simulink library "LopesDevelopmentLibrary"  (R2015b)
settings: Solver=ode45  StartTime=0.0  StopTime=10.0  RelTol=1e-3
values from neighbouring files (symbols this model uses):
  d2r = @(d) d*(pi/180)    [LopesDevelopmentLibrary_LoadParameters.m]
  ts = LopesParams.ts    [LopesDevelopmentLibrary_LoadParameters.m]
undefined symbols (not defined in the file or in its folder): anyParameterChanged, DiscIntNeverNeededParam, gcbh, LAP, LHF, LKF, LopesParams, macaddr, mxpcnetworkconfig, mxpcrtudprx, mxpcrtudptx, patientParametersChanged, port, PX, PZ, RAP, RHF, RKF, SelectorLOPESInSize, StrideTime_s, Time
undefined symbols (not defined in the file): LopesParamsSendDataArrayLen
libraries: LopesDevelopmentLibrary x327, simulink x100, dspmtrx3 x49, xpciplib x6, xpcnetworkbufferlib x5, dspsigops x4, dspstat3 x3, xpcethernetlib x2, visionstatistics x2, xpcseriallib x2, LopesDevelopmentLibraryTest x1, nmc x1
(part 2 of 12)

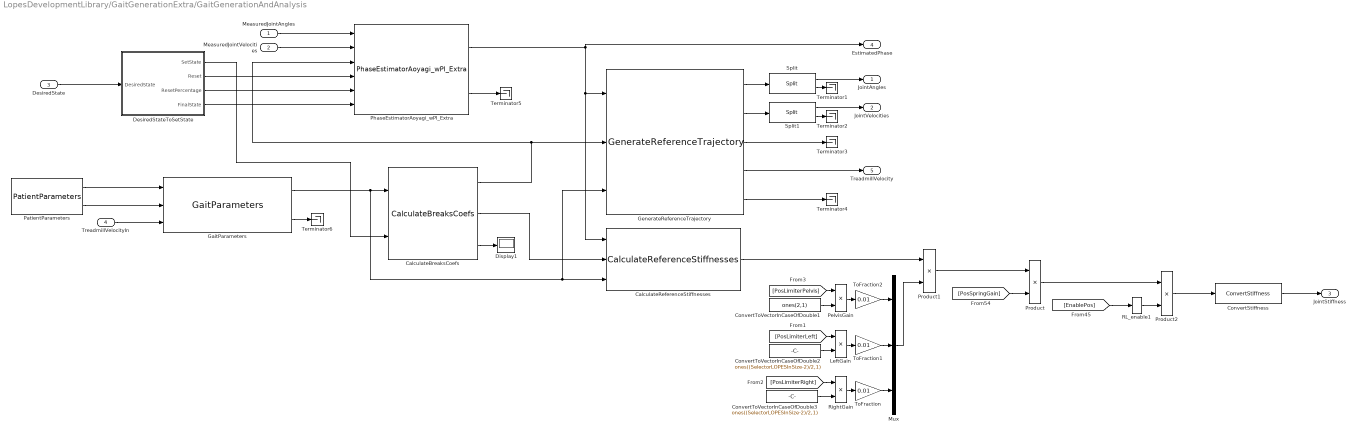
== system LopesDevelopmentLibrary/GaitGenerationExtra/GaitGenerationAndAnalysis ==
  MeasuredJointAngles : Inport
  MeasuredJointVelocities : Inport  Port=2
  DesiredState : Inport  Port=3
  TreadmillVelocityIn : Inport  Port=4
  CalculateBreaksCoefs : LopesDevelopmentLibrary/GaitGenerationExtra/CalculateBreaksCoefs
  CalculateReferenceStiffnesses : LopesDevelopmentLibrary/GaitGeneration/CalculateReferenceStiffnesses
  ConvertStiffness : LopesDevelopmentLibrary/GaitGeneration/ConvertStiffness
  ConvertToVectorInCaseOfDouble1 : Constant  Value=ones(2,1)
  ConvertToVectorInCaseOfDouble2 : Constant  Value=ones((SelectorLOPESInSize-2)/2,1)
  ConvertToVectorInCaseOfDouble3 : Constant  Value=ones((SelectorLOPESInSize-2)/2,1)
  DesiredStateToSetState : Subsystem
  Display1 : Display
  GaitParameters : LopesDevelopmentLibrary/GaitGenerationExtra/GaitParameters
  GenerateReferenceTrajectory : LopesDevelopmentLibrary/GaitGeneration/GenerateReferenceTrajectory
  LeftGain : Product
  Mux : Mux  Inputs=3
  PatientParameters : LopesDevelopmentLibrary/GaitGeneration/PatientParameters
      link override BodyLength_m: Value=1.88
      link override LowerLegLength_m: Value=0.44
      link override Mass_kg: Value=75
      link override UpperLegLength_m: Value=0.44
  PelvisGain : Product
  PhaseEstimatorAoyagi_wPI_Extra : LopesDevelopmentLibrary/GaitGenerationExtra/PhaseEstimatorAoyagi_wPI_Extra  Weights=[1.0, 0.1, 1.0, 0.1, 0.0, 0, 0.0, 0]  AoyagiFilterGain=0  AoyagiIntegralTimeConstant=5
  Product : Product
  Product1 : Product
  Product2 : Product
  RL_enable1 : nmc/RL_enable
  RightGain : Product
  Split : LopesDevelopmentLibrary/Various/Split
  Split1 : LopesDevelopmentLibrary/Various/Split
  Terminator{1..6} (6 alike) : Terminator
  ToFraction : Gain  Gain=0.01
  ToFraction1 : Gain  Gain=0.01
  ToFraction2 : Gain  Gain=0.01
  JointAngles : Outport
  JointVelocities : Outport  Port=2
  JointStiffness : Outport  Port=3
  EstimatedPhase : Outport  Port=4
  TreadmillVelocity : Outport  Port=5
  wires:
  DesiredStateToSetState/3(ResetPercentage) -> PhaseEstimatorAoyagi_wPI_Extra/5
  DesiredStateToSetState/2(Reset) -> PhaseEstimatorAoyagi_wPI_Extra/4
  DesiredState/1 -> DesiredStateToSetState/1(DesiredState)
  DesiredStateToSetState/1(SetState) -> CalculateBreaksCoefs/2
  CalculateBreaksCoefs/3 -> Display1/1
  CalculateBreaksCoefs/1 -> GenerateReferenceTrajectory/2, PhaseEstimatorAoyagi_wPI_Extra/3
  CalculateBreaksCoefs/2 -> CalculateReferenceStiffnesses/2
  PhaseEstimatorAoyagi_wPI_Extra/1 -> EstimatedPhase/1, GenerateReferenceTrajectory/1, CalculateReferenceStiffnesses/1
  GenerateReferenceTrajectory/1 -> Split/1
  Split/1 -> JointAngles/1
  Split/2 -> Terminator1/1
  GenerateReferenceTrajectory/5 -> Terminator4/1
  Split1/2 -> Terminator2/1
  PatientParameters/1 -> GaitParameters/1
  GenerateReferenceTrajectory/2 -> Split1/1
  Split1/1 -> JointVelocities/1
  MeasuredJointVelocities/1 -> PhaseEstimatorAoyagi_wPI_Extra/2
  MeasuredJointAngles/1 -> PhaseEstimatorAoyagi_wPI_Extra/1
  PhaseEstimatorAoyagi_wPI_Extra/2 -> Terminator5/1
  GenerateReferenceTrajectory/3 -> Terminator3/1
  PatientParameters/2 -> GaitParameters/2
  GaitParameters/2 -> Terminator6/1
  GaitParameters/1 -> CalculateBreaksCoefs/1, GenerateReferenceTrajectory/3, CalculateReferenceStiffnesses/3
  ConvertStiffness/1 -> JointStiffness/1
  CalculateReferenceStiffnesses/1 -> Product1/1
  [PosSpringGain] -> Product/2
  Product1/1 -> Product/1
  ConvertToVectorInCaseOfDouble1/1 -> PelvisGain/2
  [PosLimiterPelvis] -> PelvisGain/1
  [PosLimiterLeft] -> LeftGain/1
  ConvertToVectorInCaseOfDouble2/1 -> LeftGain/2
  [PosLimiterRight] -> RightGain/1
  ConvertToVectorInCaseOfDouble3/1 -> RightGain/2
  LeftGain/1 -> ToFraction1/1
  PelvisGain/1 -> ToFraction2/1
  Mux/1 -> Product1/2
  Product/1 -> Product2/1
  [EnablePos] -> RL_enable1/1
  RL_enable1/1 -> Product2/2
  Product2/1 -> ConvertStiffness/1
  RightGain/1 -> ToFraction/1
  ToFraction/1 -> Mux/3
  ToFraction1/1 -> Mux/2
  ToFraction2/1 -> Mux/1
  GenerateReferenceTrajectory/4 -> TreadmillVelocity/1
  DesiredStateToSetState/4(FinalState) -> PhaseEstimatorAoyagi_wPI_Extra/6
  TreadmillVelocityIn/1 -> GaitParameters/3

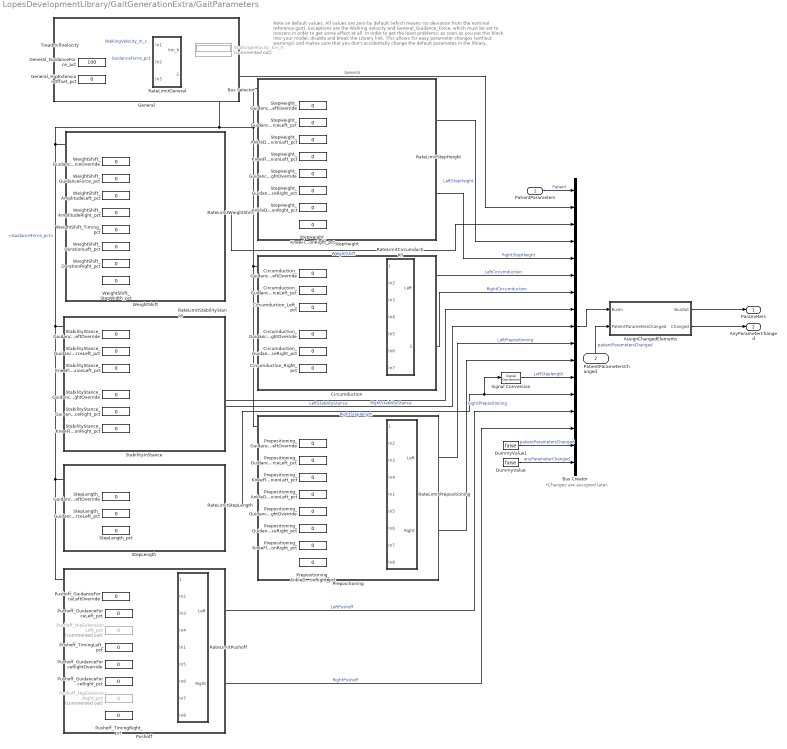
== system LopesDevelopmentLibrary/GaitGenerationExtra/GaitParameters ==
  note: Note on default values:
      | All values are zero by default (which means 'no deviation from the nominal reference gait).
      | Exceptions are the Walking velocity and General_Guidance_Force, which must be
      | set to nonzero in order to get some effect at all.
      |
      | In order to get the least problems: as soon as you put this block into your model, disable and
      | break the Library link. This allows for easy parameter changes (without warnings) and makes
      | sure that you don't accidentally change the default parametes in the library.
  note: *Changes are assigned later.
  PatientParameters : Inport
  PatientParametersChanged : Inport  Port=2
  TreadmillVelocity : Inport  Port=3
  AssignChangedElements : Subsystem
  Bus Creator : BusCreator  Inputs=17
  Bus Selector : BusSelector  OutputSignals=GuidanceForce_pct
  Circumduction : Subsystem
  Circumduction_GuidanceForceLeftOverride : Constant  Value=0  OutDataTypeStr=double
      settings: OpenFcn=|
      | b = get_param(gcb,'value');
      | if (strcmp(b,'1')),
      |   set_param (gcb,'value','0');
      | else
      |   set_param(gcb,'value','1');
      | end;
  Circumduction_GuidanceForceLeft_pct : Constant  Value=0
  Circumduction_GuidanceForceRightOverride : Constant  Value=0  OutDataTypeStr=double
      settings: OpenFcn=|
      | b = get_param(gcb,'value');
      | if (strcmp(b,'1')),
      |   set_param (gcb,'value','0');
      | else
      |   set_param(gcb,'value','1');
      | end;
  Circumduction_GuidanceForceRight_pct : Constant  Value=0
  Circumduction_Left_pct : Constant  Value=0
  Circumduction_Right_pct : Constant  Value=0
  DummyValue : Constant  Value=false  OutDataTypeStr=boolean
  DummyValue1 : Constant  Value=false
  General : Subsystem
  General_GuidanceForce_pct : Constant  Value=100
  General_HipExtensionOffset_pct : Constant  Value=0
  Prepositioning : Subsystem
  Prepositioning_AnkleDorsiFlexionLeft_pct : Constant  Value=0
  Prepositioning_AnkleDorsiFlexionRight_pct : Constant  Value=0
  Prepositioning_GuidanceForceLeftOverride : Constant  Value=0  OutDataTypeStr=double
      settings: OpenFcn=|
      | b = get_param(gcb,'value');
      | if (strcmp(b,'1')),
      |   set_param (gcb,'value','0');
      | else
      |   set_param(gcb,'value','1');
      | end;
  Prepositioning_GuidanceForceLeft_pct : Constant  Value=0
  Prepositioning_GuidanceForceRightOverride : Constant  Value=0  OutDataTypeStr=double
      settings: OpenFcn=|
      | b = get_param(gcb,'value');
      | if (strcmp(b,'1')),
      |   set_param (gcb,'value','0');
      | else
      |   set_param(gcb,'value','1');
      | end;
  Prepositioning_GuidanceForceRight_pct : Constant  Value=0
  Prepositioning_KneeFlexionLeft_pct : Constant  Value=0
  Prepositioning_KneeFlexionRight_pct : Constant  Value=0
  Pushoff : Subsystem
  Pushoff_GuidanceForceLeftOverride : Constant  Value=0  OutDataTypeStr=double
      settings: OpenFcn=|
      | b = get_param(gcb,'value');
      | if (strcmp(b,'1')),
      |   set_param (gcb,'value','0');
      | else
      |   set_param(gcb,'value','1');
      | end;
  Pushoff_GuidanceForceLeft_pct : Constant  Value=0
  Pushoff_GuidanceForceRightOverride : Constant  Value=0  OutDataTypeStr=double
      settings: OpenFcn=|
      | b = get_param(gcb,'value');
      | if (strcmp(b,'1')),
      |   set_param (gcb,'value','0');
      | else
      |   set_param(gcb,'value','1');
      | end;
  Pushoff_GuidanceForceRight_pct : Constant  Value=0
  Pushoff_HipExtensioRight_pct : Constant  Commented=on  Value=0
  Pushoff_HipExtensionLeft_pct : Constant  Commented=on  Value=0
  Pushoff_TimingLeft_pct : Constant  Value=0
  Pushoff_TimingRight_pct : Constant  Value=0
  RateLimitCircumduction : Subsystem
  RateLimitGeneral : Subsystem
  RateLimitPrepositioning : Subsystem
  RateLimitPushoff : Subsystem
  RateLimitStabilityStance : Subsystem
  RateLimitStepHeight : Subsystem
  RateLimitStepLength : Subsystem
  RateLimitWeightShift : Subsystem
  Signal Conversion : SignalConversion
  StabilityInStance : Subsystem
  StabilityStance_GuidanceForceLeftOverride : Constant  Value=0  OutDataTypeStr=double
      settings: OpenFcn=|
      | b = get_param(gcb,'value');
      | if (strcmp(b,'1')),
      |   set_param (gcb,'value','0');
      | else
      |   set_param(gcb,'value','1');
      | end;
  StabilityStance_GuidanceForceLeft_pct : Constant  Value=0
  StabilityStance_GuidanceForceRightOverride : Constant  Value=0  OutDataTypeStr=double
      settings: OpenFcn=|
      | b = get_param(gcb,'value');
      | if (strcmp(b,'1')),
      |   set_param (gcb,'value','0');
      | else
      |   set_param(gcb,'value','1');
      | end;
  StabilityStance_GuidanceForceRight_pct : Constant  Value=0
  StabilityStance_KneeFlexionLeft_pct : Constant  Value=0
  StabilityStance_KneeFlexionRight_pct : Constant  Value=0
  StepHeight : Subsystem
  StepHeight_AnkleDorsiflexionLeft_pct : Constant  Value=0
  StepHeight_AnkleDorsiflexionRight_pct : Constant  Value=0
  StepHeight_GuidanceForceLeftOverride : Constant  Value=0  OutDataTypeStr=double
      settings: OpenFcn=|
      | b = get_param(gcb,'value');
      | if (strcmp(b,'1')),
      |   set_param (gcb,'value','0');
      | else
      |   set_param(gcb,'value','1');
      | end;
  StepHeight_GuidanceForceLeft_pct : Constant  Value=0
  StepHeight_GuidanceForceRightOverride : Constant  Value=0  OutDataTypeStr=double
      settings: OpenFcn=|
      | b = get_param(gcb,'value');
      | if (strcmp(b,'1')),
      |   set_param (gcb,'value','0');
      | else
      |   set_param(gcb,'value','1');
      | end;
  StepHeight_GuidanceForceRight_pct : Constant  Value=0
  StepHeight_KneeFlexionLeft_pct : Constant  Value=0
  StepHeight_KneeFlexionRight_pct : Constant  Value=0
  StepLength : Subsystem
  StepLength_GuidanceForceLeftOverride : Constant  Value=0  OutDataTypeStr=double
      settings: OpenFcn=|
      | b = get_param(gcb,'value');
      | if (strcmp(b,'1')),
      |   set_param (gcb,'value','0');
      | else
      |   set_param(gcb,'value','1');
      | end;
  StepLength_GuidanceForceLeft_pct : Constant  Value=0
  StepLength_pct : Constant  Value=0
  WalkingVelocity_km_h : Display  Commented=on
  WeightShift : Subsystem
  WeightShift_AmplitudeLeft_pct : Constant  Value=0
  WeightShift_AmplitudeRight_pct : Constant  Value=0
  WeightShift_DurationLeft_pct : Constant  Value=0
  WeightShift_DurationRight_pct : Constant  Value=0
  WeightShift_GuidanceForceOverride : Constant  Value=0  OutDataTypeStr=double
      settings: OpenFcn=|
      | b = get_param(gcb,'value');
      | if (strcmp(b,'1')),
      |   set_param (gcb,'value','0');
      | else
      |   set_param(gcb,'value','1');
      | end;
  WeightShift_GuidanceForce_pct : Constant  Value=0
  WeightShift_StepWidth_pct : Constant  Value=0
  WeightShift_Timing_pct : Constant  Value=0
  Parameters : Outport
  AnyParameterChanged : Outport  Port=2
  wires:
  AssignChangedElements/1(BusOut) -> Parameters/1
  Signal Conversion/1 -> Bus Creator/12  "LeftSteplength"
  DummyValue1/1 -> Bus Creator/16  "patientParametersChanged"
  DummyValue/1 -> Bus Creator/17  "anyParameterChanged"
  RateLimitWeightShift/1(Out1) -> Bus Creator/3  "WeightShift"
  PatientParameters/1 -> Bus Creator/1  "Patient"
  RateLimitStepHeight/1(Left) -> Bus Creator/4  "LeftStepHeight"
  RateLimitStepHeight/2(Right) -> Bus Creator/5  "RightStepHeight"
  RateLimitStabilityStance/1(Left) -> Bus Creator/8  "LeftStabilityStance"
  RateLimitStabilityStance/2(Right) -> Bus Creator/9  "RightStabilityStance"
  RateLimitPrepositioning/1(Left) -> Bus Creator/10  "LeftPrepositioning"
  RateLimitPrepositioning/2(Right) -> Bus Creator/11  "RightPrepositioning"
  RateLimitStepLength/1(StepLength) -> Bus Creator/13, Signal Conversion/1  "RightSteplength"
  RateLimitCircumduction/1(Left) -> Bus Creator/6  "LeftCircumduction"
  RateLimitCircumduction/2(Right) -> Bus Creator/7  "RightCircumduction"
  WeightShift_GuidanceForceOverride/1 -> RateLimitWeightShift/2(In2)
  WeightShift_GuidanceForce_pct/1 -> RateLimitWeightShift/3(In3)
  WeightShift_AmplitudeLeft_pct/1 -> RateLimitWeightShift/4(In4)
  WeightShift_AmplitudeRight_pct/1 -> RateLimitWeightShift/5(In5)
  WeightShift_Timing_pct/1 -> RateLimitWeightShift/6(In6)
  WeightShift_DurationLeft_pct/1 -> RateLimitWeightShift/7(In7)
  WeightShift_DurationRight_pct/1 -> RateLimitWeightShift/8(In8)
  WeightShift_StepWidth_pct/1 -> RateLimitWeightShift/9(In9)
  StepHeight_GuidanceForceLeftOverride/1 -> RateLimitStepHeight/2(In2)
  StepHeight_GuidanceForceLeft_pct/1 -> RateLimitStepHeight/3(In3)
  StepHeight_KneeFlexionLeft_pct/1 -> RateLimitStepHeight/5(In4)
  StepHeight_GuidanceForceRightOverride/1 -> RateLimitStepHeight/6(In5)
  StepHeight_GuidanceForceRight_pct/1 -> RateLimitStepHeight/7(In6)
  StepHeight_KneeFlexionRight_pct/1 -> RateLimitStepHeight/9(In7)
  Circumduction_GuidanceForceLeftOverride/1 -> RateLimitCircumduction/2(In2)
  Circumduction_GuidanceForceLeft_pct/1 -> RateLimitCircumduction/3(In3)
  Circumduction_Left_pct/1 -> RateLimitCircumduction/4(In4)
  Circumduction_GuidanceForceRightOverride/1 -> RateLimitCircumduction/5(In5)
  Circumduction_GuidanceForceRight_pct/1 -> RateLimitCircumduction/6(In6)
  Circumduction_Right_pct/1 -> RateLimitCircumduction/7(In7)
  StabilityStance_GuidanceForceLeftOverride/1 -> RateLimitStabilityStance/2(In2)
  StabilityStance_GuidanceForceLeft_pct/1 -> RateLimitStabilityStance/3(In3)
  StabilityStance_KneeFlexionLeft_pct/1 -> RateLimitStabilityStance/4(In4)
  StabilityStance_GuidanceForceRightOverride/1 -> RateLimitStabilityStance/5(In5)
  StabilityStance_GuidanceForceRight_pct/1 -> RateLimitStabilityStance/6(In6)
  StabilityStance_KneeFlexionRight_pct/1 -> RateLimitStabilityStance/7(In7)
  Prepositioning_GuidanceForceLeftOverride/1 -> RateLimitPrepositioning/2(In2)
  Prepositioning_GuidanceForceLeft_pct/1 -> RateLimitPrepositioning/3(In3)
  Prepositioning_KneeFlexionLeft_pct/1 -> RateLimitPrepositioning/4(In4)
  Prepositioning_GuidanceForceRightOverride/1 -> RateLimitPrepositioning/6(In5)
  Prepositioning_GuidanceForceRight_pct/1 -> RateLimitPrepositioning/7(In6)
  Prepositioning_KneeFlexionRight_pct/1 -> RateLimitPrepositioning/8(In7)
  StepLength_GuidanceForceLeftOverride/1 -> RateLimitStepLength/2(In2)
  StepLength_GuidanceForceLeft_pct/1 -> RateLimitStepLength/3(In3)
  StepLength_pct/1 -> RateLimitStepLength/4(In4)
  Bus Selector/1 -> RateLimitStepHeight/1(GeneralGF), RateLimitPrepositioning/1(GeneralGF), RateLimitCircumduction/1(GeneralGF), RateLimitWeightShift/1(GeneralGF), RateLimitPushoff/1(GeneralGF), RateLimitStepLength/1(GeneralGF), RateLimitStabilityStance/1(GeneralGF)  "<GuidanceForce_pct>"
  RateLimitGeneral/2(General) -> Bus Creator/2, Bus Selector/1  "General"
  TreadmillVelocity/1 -> RateLimitGeneral/1(In1)  "WalkingVelocity_m_s"
  General_GuidanceForce_pct/1 -> RateLimitGeneral/2(In2)  "GuidanceForce_pct"
  General_HipExtensionOffset_pct/1 -> RateLimitGeneral/3(In3)
  RateLimitGeneral/1(km_h) -> WalkingVelocity_km_h/1
  Bus Creator/1 -> AssignChangedElements/1(BusIn)
  PatientParametersChanged/1 -> AssignChangedElements/2(PatientParametersChanged)  "patientParametersChanged"
  AssignChangedElements/2(Changed) -> AnyParameterChanged/1
  StepHeight_AnkleDorsiflexionLeft_pct/1 -> RateLimitStepHeight/4(In1)
  StepHeight_AnkleDorsiflexionRight_pct/1 -> RateLimitStepHeight/8(In8)
  Prepositioning_AnkleDorsiFlexionLeft_pct/1 -> RateLimitPrepositioning/5(In1)
  Prepositioning_AnkleDorsiFlexionRight_pct/1 -> RateLimitPrepositioning/9(In8)
  Pushoff_GuidanceForceLeft_pct/1 -> RateLimitPushoff/3(In3)
  Pushoff_HipExtensionLeft_pct/1 -> RateLimitPushoff/4(In4)
  Pushoff_GuidanceForceRightOverride/1 -> RateLimitPushoff/6(In5)
  Pushoff_GuidanceForceRight_pct/1 -> RateLimitPushoff/7(In6)
  Pushoff_HipExtensioRight_pct/1 -> RateLimitPushoff/8(In7)
  Pushoff_TimingLeft_pct/1 -> RateLimitPushoff/5(In1)
  Pushoff_TimingRight_pct/1 -> RateLimitPushoff/9(In8)
  RateLimitPushoff/1(Left) -> Bus Creator/14  "LeftPushoff"
  RateLimitPushoff/2(Right) -> Bus Creator/15  "RightPushoff"
  Pushoff_GuidanceForceLeftOverride/1 -> RateLimitPushoff/2(In2)

== system LopesDevelopmentLibrary/GaitGenerationExtra/PhaseEstimatorAoyagi_wPI_Extra ==
  note: This block is a phase estimator based on the paper by Aoyagi 2007. It consists of two parts:
      | -  a raw estimator which estimates the current phase simply based on the euclidean distance
      |    to each point on the trajectory (it returns the phase at which this distance is minimum), and
      | - a (sort-of-low-pass)-filter which generates a continuous and not-too-fast-changing output phase.
  MeasuredJointAngles : Inport
  MeasuredJointVelocities : Inport  Port=2
  BreaksCoefs : Inport  Port=3
  ResetHighActive : Inport  Port=4
  X0 : Inport  Port=5
  FinalState : Inport  Port=6
  Bus Selector : BusSelector  OutputSignals=StrideTime_s
  EstimatePhaseDirectlyAoyagi : Subsystem
  PhaseFilterAoyagi : Subsystem
  EstmiatedPhase_pct : Outport
  EstmiatedPhaseRate_pct_s : Outport  Port=2
  wires:
  FinalState/1 -> PhaseFilterAoyagi/5(FinalState)
  X0/1 -> PhaseFilterAoyagi/4(x0)
  MeasuredJointAngles/1 -> EstimatePhaseDirectlyAoyagi/1(MeasuredJointAngles)
  BreaksCoefs/1 -> EstimatePhaseDirectlyAoyagi/3(BreaksCoefs), Bus Selector/1
  MeasuredJointVelocities/1 -> EstimatePhaseDirectlyAoyagi/2(MeasuredJointVelocities)
  EstimatePhaseDirectlyAoyagi/1(EstimtatedPhaseUnfiltered) -> PhaseFilterAoyagi/1(EstimatedPhaseUnfiltered)
  Bus Selector/1 -> PhaseFilterAoyagi/2(ReferenceStrideTime)  "<StrideTime_s>"
  PhaseFilterAoyagi/1(EstimatedPhase) -> EstmiatedPhase_pct/1
  ResetHighActive/1 -> PhaseFilterAoyagi/3(ResetHighActive)
  PhaseFilterAoyagi/2(EstimatedPhaseRate) -> EstmiatedPhaseRate_pct_s/1

== system LopesDevelopmentLibrary/GaitGenerationExtra/VelocityHold ==
  SetState : Inport
  InputState : Inport  Port=2
  VeloIn : Inport  Port=3  OutDataTypeStr=double
  Compare To Constant5 : simulink/Logic and Bit Operations/Compare To Constant  Commented=on  relop===  const=3.0  OutDataTypeStr=boolean
  Compare To Constant6 : simulink/Logic and Bit Operations/Compare To Constant  Commented=on  relop=~=  const=301  OutDataTypeStr=boolean
  Compare To Constant7 : simulink/Logic and Bit Operations/Compare To Constant  Commented=on  relop=~=  const=302  OutDataTypeStr=boolean
  Compare To Constant8 : simulink/Logic and Bit Operations/Compare To Constant  Commented=on  relop=~=  const=401  OutDataTypeStr=boolean
  Compare To Constant9 : simulink/Logic and Bit Operations/Compare To Constant  Commented=on  relop=~=  const=402  OutDataTypeStr=boolean
  Constant : Constant  Value=0.25
  KeepSpeedUntillStopState : Gain  Commented=on  Gain=0.25
  Logical Operator2 : Logic  Commented=on  Inputs=4  AllPortsSameDT=off  OutDataTypeStr=boolean
  Logical Operator3 : Logic  Commented=on  AllPortsSameDT=off  OutDataTypeStr=boolean
  MATLAB Function : MATLAB Function  TreatAsAtomicUnit=on
      settings: MinAlgLoopOccurrences=on
  VeloOut : Outport  PortDimensions=1
  wires:
  SetState/1 -> MATLAB Function/2(SetState)
  Compare To Constant5/1 -> Logical Operator3/1
  Compare To Constant7/1 -> Logical Operator2/2
  ? -> Compare To Constant5/1
  Compare To Constant9/1 -> Logical Operator2/4
  Logical Operator2/1 -> Logical Operator3/2
  Compare To Constant6/1 -> Logical Operator2/1
  Compare To Constant8/1 -> Logical Operator2/3
  Logical Operator3/1 -> KeepSpeedUntillStopState/1
  ? -> Compare To Constant6/1
  ? -> Compare To Constant7/1
  ? -> Compare To Constant8/1
  ? -> Compare To Constant9/1
  InputState/1 -> MATLAB Function/1(InputState)
  Constant/1 -> MATLAB Function/4(LowerBound)
  MATLAB Function/1(VeloOut) -> VeloOut/1
  VeloIn/1 -> MATLAB Function/3(VeloIn)

== system LopesDevelopmentLibrary/GaitPhaseDetection/Gait Phase Detection with Wrapper ==
  note: Phase:
      | -2 -> Flight (or probably error)
      | -1 -> Error
      | 0 -> Error
      | 1 -> Double stance, left in front
      | 2 -> Right swing
      | 3 -> Double stance, right in front
      | 4 -> Left swing
  Cartesian Positions : Inport
  Treadmill : Inport  Port=2
  Data selection : Subsystem
  LeftLegWalking : Subsystem
  No speed detection : Subsystem
  Phase_selection : Subsystem
  RightLegWalking : Subsystem
  Smart derivative : Subsystem
  wAnkleConvert : Selector  InputPortWidth=33  IndexOptions=Index vector (dialog)  Indices=[1:12 19:27]  OutputSizes=1
  Phase : Outport
  wires:
  No speed detection/3(Right) -> Phase_selection/7(RightStop)
  No speed detection/2(Left) -> Phase_selection/6(LeftStop)
  Cartesian Positions/1 -> wAnkleConvert/1
  Phase_selection/1(Phase) -> Phase/1
  Smart derivative/4(ankle_y_r_dot) -> RightLegWalking/1(ankle_y_r_dot)
  Smart derivative/5(ankle_x_r_dot) -> RightLegWalking/2(ankle_x_r_dot)
  Smart derivative/6(angle_knee_r_dot) -> RightLegWalking/3(knee_angle_dot)
  Data selection/3(angle_knee_l) -> Smart derivative/3(angle_knee_l)
  Data selection/6(angle_knee_r) -> Smart derivative/6(angle_knee_r)
  Data selection/4(ankle_y_r) -> Smart derivative/4(ankle_y_r)
  Data selection/5(ankle_x_r) -> Phase_selection/5(ankle_x_r), Smart derivative/5(ankle_x_r)
  Data selection/2(ankle_x_l) -> Phase_selection/4(ankle_x_l), Smart derivative/2(ankle_x_l)
  Data selection/1(ankle_y_l) -> Smart derivative/1(ankle_y_l)
  Smart derivative/3(angle_knee_l_dot) -> LeftLegWalking/3(knee_angle_dot)
  Smart derivative/2(ankle_x_l_dot) -> LeftLegWalking/2(ankle_x_r_dot)
  Smart derivative/1(ankle_y_l_dot) -> LeftLegWalking/1(ankle_y_r_dot)
  Treadmill/1 -> Data selection/2(Treadmill), No speed detection/3(Treadmill)
  No speed detection/1(gaitSwitch) -> Phase_selection/3(Gait_switch)
  LeftLegWalking/1(Left) -> Phase_selection/1(LeftWalking)
  RightLegWalking/1(right) -> Phase_selection/2(RightWalking)
  Data selection/7(Treadmill speed) -> Smart derivative/7(treadmill speed), No speed detection/1(curVel), LeftLegWalking/4(belt_speed), RightLegWalking/4(belt_speed)
  wAnkleConvert/1 -> Data selection/1(Cart_pos), No speed detection/2(CartesianPositions)

== system LopesDevelopmentLibrary/GaitPhaseDetection/Gait Phase detection ==
  note: Phase:
      | -1 -> Error
      | 0 -> Error
      | 1 -> Double stance, left in front
      | 2 -> Right swing
      | 3 -> Double stance, right in front
      | 4 -> Left swing
  Cartesian Positions : Inport
  Treadmill : Inport  Port=2
  Data selection : Subsystem
  LeftLeg : Subsystem
  No speed detection : Subsystem
  Phase_selection : Subsystem
  RightLeg : Subsystem
  Smart derivative : Subsystem
  phase : Outport
  wires:
  Smart derivative/4(ankle_y_r_dot) -> RightLeg/1(ankle_y_r_dot)
  Smart derivative/5(ankle_x_r_dot) -> RightLeg/2(ankle_x_r_dot)
  Smart derivative/6(angle_knee_r_dot) -> RightLeg/3(knee_angle_dot)
  Data selection/7(Treadmill speed) -> Smart derivative/7(treadmill speed), No speed detection/1(curVel), LeftLeg/4(belt_speed), RightLeg/4(belt_speed)
  Data selection/3(angle_knee_l) -> Smart derivative/3(angle_knee_l)
  Data selection/6(angle_knee_r) -> Smart derivative/6(angle_knee_r)
  Data selection/4(ankle_y_r) -> Smart derivative/4(ankle_y_r)
  Data selection/5(ankle_x_r) -> Smart derivative/5(ankle_x_r), Phase_selection/5(ankle_x_r)
  Data selection/2(ankle_x_l) -> Smart derivative/2(ankle_x_l), Phase_selection/4(ankle_x_l)
  Data selection/1(ankle_y_l) -> Smart derivative/1(ankle_y_l)
  Smart derivative/3(angle_knee_l_dot) -> LeftLeg/3(knee_theta_l_dot)
  Smart derivative/2(ankle_x_l_dot) -> LeftLeg/2(ankle_x_l_dot)
  Smart derivative/1(ankle_y_l_dot) -> LeftLeg/1(ankle_y_l_dot)
  Treadmill/1 -> Data selection/2(Treadmill)
  Cartesian Positions/1 -> Data selection/1(Cart_pos)
  Phase_selection/1(Phase) -> phase/1
  No speed detection/1(gaitSwitch) -> Phase_selection/3(Gait_switch)
  LeftLeg/1(left) -> Phase_selection/1(Left)
  RightLeg/1(right) -> Phase_selection/2(Right)

== system LopesDevelopmentLibrary/Mindwalker/Mindwalker_AdaptiveTreadmillVelocity ==
  note: The treadmill should, on average, have the same velocity as the resulting
      | walking velocity (keeping in mind that the user regularly stands still). We do this
      | by making the treadmill velocity a function of PX: the more to the front the
      | user is, the faster the treadmill goes. In order to get everything smooth, we also use
      | a (very low frequency) low pas filter. The aim is that, you'll never be pushed against the
      | back stop of PX by the treadmill if you stand still. Therefore, we have a 'dead zone'
      | close to the back stop, where the treadmill is off. Outside the dead zone, the
      | velocity is linear with PX, up to a maximum of V_treadmill_max, which is the velocity
      | if you'd initiate steps as fast as possible. The boundary between dead zone and linear zone is
      | called 'Threshold'.
      |
      | Note that the (current) range of motion for PX is -0.18...0.17 m.
  Lopes_ModelPos : Inport
  State : Inport  Port=2
  CalculateThreshold : Sum
  CompareAny : LopesDevelopmentLibrary/Various/CompareAny  values=[2,3,5,6,8,9]
  Data Type Conversion : DataTypeConversion  OutDataTypeStr=double
  Demux : Demux  Outputs=2
  Divide : Product  Inputs=*/
  GetPX : Selector  InputPortWidth=11  IndexOptions=Index vector (dialog)  Indices=1  OutputSizes=1
  Product : Product  RndMeth=Zero
  Product1 : Product  RndMeth=Zero
  RangeOfMotionPX_m : Constant  Value=[-0.18,0.17]
  Saturation : Saturate  UpperLimit=5  LowerLimit=0
  SecondOrderLowPassFilter : LopesDevelopmentLibrary/Various/SecondOrderLowPassFilter  w=10*(2*pi)  z=1
  Subtract : Sum  Inputs=+-
  Subtract1 : Sum  Inputs=+-
  V_treadmill_max : Constant  Value=0.5
  deadZone_m : Constant  Value=0.01
  TreadmillVelocity : Outport
  wires:
  Saturation/1 -> TreadmillVelocity/1
  Data Type Conversion/1 -> Product1/2
  State/1 -> CompareAny/1
  CompareAny/1 -> Data Type Conversion/1
  Product1/1 -> Product/2
  SecondOrderLowPassFilter/1 -> Saturation/1
  Product/1 -> SecondOrderLowPassFilter/1
  V_treadmill_max/1 -> Product1/1
  Divide/1 -> Product/1
  Subtract1/1 -> Divide/2
  Subtract/1 -> Divide/1
  Lopes_ModelPos/1 -> GetPX/1
  CalculateThreshold/1 -> Subtract1/2, Subtract/2
  Demux/1 -> CalculateThreshold/2
  deadZone_m/1 -> CalculateThreshold/1
  Demux/2 -> Subtract1/1
  RangeOfMotionPX_m/1 -> Demux/1
  GetPX/1 -> Subtract/1

== system LopesDevelopmentLibrary/Mindwalker/Mindwalker_Lopes_Conversion ==
  note: Visualization works only in normal
      | simulation mode (not when using xPC Target)
  Lopes_ModelPos : Inport
  Lopes_ModelVel : Inport  Port=2
  MW_SpringPositions : Inport  Port=3
  MW_SpringVelocities : Inport  Port=4
  MW_SpringStiffnesses : Inport  Port=5
  MW_BiasForces : Inport  Port=6
  CalculateForceOnTorso : Subsystem
  EnableVisualization : Constant  OutDataTypeStr=double
      settings: OpenFcn=|
      | b = get_param(gcb,'value');
      | if (strcmp(b,'1')),
      |   set_param (gcb,'value','0');
      | else
      |   set_param(gcb,'value','1');
      | end;
  ITorso_kgm2 : Constant  Value=6.73
  LopesToMWPosition : Subsystem
  LopesToMWVelocity : Subsystem
  MWToLopesPosition : Subsystem
  MWToLopesVelocity : Subsystem
  Mux1 : Mux  Inputs=2
  Mux2 : Mux  Inputs=2
  TorsoDynamics : Subsystem
  VisualizeStickFigure : Subsystem  Commented=on
  Zeros : Constant  Value=[0;0]
  Zeros1 : Constant  Value=[0,0]
  Lopes_SpringPositions : Outport
  Lopes_SpringVelocities : Outport  Port=2
  Lopes_SpringStiffnesses : Outport  Port=3
  Lopes_BiasForces : Outport  Port=4
  MW_ModelPos : Outport  Port=5
  MW_ModelVel : Outport  Port=6
  wires:
  LopesToMWVelocity/1(MW_Joints) -> MW_ModelVel/1
  LopesToMWPosition/1(MW_Joints) -> MW_ModelPos/1
  CalculateForceOnTorso/1(ForceOnTorso) -> TorsoDynamics/1(Force)
  Lopes_ModelVel/1 -> LopesToMWVelocity/1(Lopes_Joints), CalculateForceOnTorso/6(Lopes_ModelVel)
  TorsoDynamics/2(TorsoFlexionVelocity) -> MWToLopesVelocity/2(TorsoValue), LopesToMWVelocity/2(TorsoValue)
  TorsoDynamics/1(TorsoFlexion) -> VisualizeStickFigure/1(TorsoFlexion), MWToLopesPosition/2(TorsoValue), LopesToMWPosition/2(TorsoValue)
  EnableVisualization/1 -> VisualizeStickFigure/3(Enable)
  MW_BiasForces/1 -> CalculateForceOnTorso/4(MW_BiasForces), Mux1/2
  Mux2/1 -> Lopes_SpringStiffnesses/1
  MW_SpringPositions/1 -> MWToLopesPosition/1(RelativeJoints)
  Zeros/1 -> Mux1/1
  Zeros1/1 -> Mux2/1
  Lopes_ModelPos/1 -> CalculateForceOnTorso/5(Lopes_ModelPos), VisualizeStickFigure/2(Lopes_ModelPos), LopesToMWPosition/1(Lopes_Joints)
  MWToLopesPosition/1(AbsoluteJoints) -> Lopes_SpringPositions/1, CalculateForceOnTorso/1(MW_SpringPositions)
  MWToLopesVelocity/1(AbsoluteJoints) -> Lopes_SpringVelocities/1, CalculateForceOnTorso/2(MW_SpringVelocities)
  MW_SpringVelocities/1 -> MWToLopesVelocity/1(RelativeJoints)
  ITorso_kgm2/1 -> CalculateForceOnTorso/7(Inertia), TorsoDynamics/2(Inertia)
  MW_SpringStiffnesses/1 -> Mux2/2, CalculateForceOnTorso/3(MW_SpringStiffness)
  Mux1/1 -> Lopes_BiasForces/1

== system LopesDevelopmentLibrary/Robot control blocks/FromLopes ==
  note: These gains are here to have a common
      | location from where we can obtain the
      | values, for example by using the
      | xpc module in Python.
  note: This block periodically (with a period of Decimation*sampletime) requests joint angle
      | data from the LLC. This happens by sending a request string, and receiving the
      | response from the LLC. Note that it may be the case that it will receive old data
      | (this happens when the LLC was not fast enough to process the request, which may happen
      | if the receive block is executed very shortly after the sending block). So, it could be
      | that the received data is (Decimation*sampletime) seconds old.
  note: If ErrorValue is zero, everything is fine. If nonzero,
      | refer to the code inside ParseString to see
      | what's wrong.
  AnalogInput_ : Concatenate  NumInputs=1
  CartesianPositions_ : Concatenate  NumInputs=1
  Decimation : LopesDevelopmentLibrary/Various/Decimation
  EnableAnalogInput : Constant  OutDataTypeStr=double
      settings: OpenFcn=|
      | b = get_param(gcb,'value');
      | if (strcmp(b,'1')),
      |   set_param (gcb,'value','0');
      | else
      |   set_param(gcb,'value','1');
      | end;
  EnableDebugStringsInMatlab : Constant  Value=0  OutDataTypeStr=double
      settings: OpenFcn=|
      | b = get_param(gcb,'value');
      | if (strcmp(b,'1')),
      |   set_param (gcb,'value','0');
      | else
      |   set_param(gcb,'value','1');
      | end;
  ErrorValue : Display  Commented=on
      settings: AttributesFormatString=%<Tag>
  GenerateString : Subsystem
  LLCReceiveUDPChannel2 : LopesDevelopmentLibrary/BlocksForInternalUse/LLC Communication/LLCReceiveUDP  port=LopesParams.Communication.channel2ReceivePort
  LLCSendUDPChannel2 : LopesDevelopmentLibrary/BlocksForInternalUse/LLC Communication/LLCSendUDP  port=LopesParams.Communication.channel2SendPort
  Logical Operator : Logic  AllPortsSameDT=off  OutDataTypeStr=boolean
  Logical Operator1 : Logic  AllPortsSameDT=off  OutDataTypeStr=boolean
  MeasForces_ : Concatenate  NumInputs=1
  MeasPos_ : Concatenate  NumInputs=1
  ModelAcc_ : Concatenate  NumInputs=1
  ModelPos_ : Concatenate  NumInputs=1
  ModelVel_ : Concatenate  NumInputs=1
  One : Constant
  ParseError_ : Concatenate  NumInputs=1
  ParseString : Subsystem
  PreRecv : Constant  Value=uint8(['FromLopes Recv: '])
  PreSend : Constant  Value=uint8(['FromLopes Send: '])
  ShowStringInMatlabConsole : MATLAB Function  TreatAsAtomicUnit=on
  ShowStringInMatlabConsole1 : MATLAB Function  TreatAsAtomicUnit=on
  Treadmill_ : Concatenate  NumInputs=1
  ~Debug : Subsystem
      mask Display: disp('')
  Error : Outport
  ModelPos : Outport  Port=2
  ModelVel : Outport  Port=3
  ModelAcc : Outport  Port=4
  MeasPos : Outport  Port=5
  MeasForces : Outport  Port=6
  CartesianPositions : Outport  Port=7
  Treadmill : Outport  Port=8
  AnalogInput : Outport  Port=9
  wires:
  AnalogInput_/1 -> AnalogInput/1
  ParseString/9(AnalogInput) -> AnalogInput_/1
  EnableAnalogInput/1 -> GenerateString/1(EnableAnaloginput)
  PreSend/1 -> ShowStringInMatlabConsole1/3(pre)
  GenerateString/2(s_len) -> ShowStringInMatlabConsole1/2(len), LLCSendUDPChannel2/2
  GenerateString/1(s) -> ShowStringInMatlabConsole1/1(stringArray), LLCSendUDPChannel2/1
  Treadmill_/1 -> Treadmill/1
  CartesianPositions_/1 -> CartesianPositions/1
  MeasForces_/1 -> MeasForces/1
  MeasPos_/1 -> MeasPos/1
  ModelAcc_/1 -> ModelAcc/1
  ModelVel_/1 -> ModelVel/1
  ModelPos_/1 -> ModelPos/1
  ParseError_/1 -> ErrorValue/1, Error/1
  ParseString/8(Treadmill) -> Treadmill_/1
  ParseString/7(ModelCartPos) -> CartesianPositions_/1
  ParseString/6(MeasForce) -> MeasForces_/1
  ParseString/4(ModelAcc) -> ModelAcc_/1
  ParseString/3(ModelVel) -> ModelVel_/1
  ParseString/2(ModelPos) -> ModelPos_/1
  ParseString/1(ParseError) -> ParseError_/1
  ParseString/5(MeasPos) -> MeasPos_/1
  Decimation/1 -> Logical Operator/2, LLCSendUDPChannel2/Enable, GenerateString/Enable
  PreRecv/1 -> ShowStringInMatlabConsole/3(pre)
  LLCReceiveUDPChannel2/2 -> ParseString/2(In2), ShowStringInMatlabConsole/2(len)
  LLCReceiveUDPChannel2/1 -> ShowStringInMatlabConsole/1(stringArray), ParseString/1(In1)
  EnableDebugStringsInMatlab/1 -> Logical Operator1/1, Logical Operator/1
  Logical Operator/1 -> ShowStringInMatlabConsole1/4(enable)
  One/1 -> ParseString/Enable, LLCReceiveUDPChannel2/Enable, Logical Operator1/2
  Logical Operator1/1 -> ShowStringInMatlabConsole/4(enable)

== system LopesDevelopmentLibrary/Robot control blocks/GeneralLopes ==
  note: 0: off
      | 1: init
      | 2: home
      | 3: stop
      | 4: position
      | 5: force
  note: 0: off
      | 1: init
      | 2: home
      | 3: stop
      | 4: position
      | 5: force
  note: This block periodically (with a period of Decimation*sampletime) checks the state of Lopes.
      | Additionally, it allows the user to request a state ('off', 'init', 'home', 'stop','position', 'force').
      | This happens by sending a request string, and receiving the
      | response from the LLC. Note that it may be the case that it will receive old data
      | (this happens when the LLC was not fast enough to process the request, which may happen
      | if the receive block is executed very shortly after the sending block).
  note: These blocks are here to have a common
      | location from where we can obtain the
      | values, for example by using the
      | xpc module in Python.
  note: You can leave this input
      | unconnected to get the
      | default inertia
  note: Set to 0 to disable
      | the watchdog
  note: -1: No message received (note that if decimation~=1, this happens  often)
      | 0: No error
      | 1: Error
  note: Temporarily removed input
      | SegmentInertia because it
      | doesn't affect the used inertia
      | (LLC uses CartesianInertia by default)
  DesiredState : Inport
  AnyMessageWasReceived : Subsystem
  Bus Creator : BusCreator  Inputs=6
  Decimation : LopesDevelopmentLibrary/Various/Decimation
      settings: Decimation=10
  EnableDebugStringsInMatlab : Constant  Value=0  OutDataTypeStr=double
      settings: OpenFcn=|
      | b = get_param(gcb,'value');
      | if (strcmp(b,'1')),
      |   set_param (gcb,'value','0');
      | else
      |   set_param(gcb,'value','1');
      | end;
  ErrorDisplay : Display  Commented=on
      settings: AttributesFormatString=%<Tag>
  GenerateString : Subsystem
  Ground : Ground
  LLC Network Configuration : LopesDevelopmentLibrary/BlocksForInternalUse/LLC Communication/LLC Network Configuration
  LLCReceiveUDPChannel1 : LopesDevelopmentLibrary/BlocksForInternalUse/LLC Communication/LLCReceiveUDP  port=LopesParams.Communication.channel1ReceivePort
  LLCSendUDPChannel1 : LopesDevelopmentLibrary/BlocksForInternalUse/LLC Communication/LLCSendUDP  port=LopesParams.Communication.channel1SendPort
  Logical Operator : Logic  AllPortsSameDT=off  OutDataTypeStr=boolean
  Logical Operator1 : Logic  AllPortsSameDT=off  OutDataTypeStr=boolean
  One : Constant
  ParseString : Subsystem
  PreRecv : Constant  Value=uint8(['General Recv: '])
  PreSend : Constant  Value=uint8(['General Send: '])
  ShowStringInMatlabConsole : MATLAB Function  TreatAsAtomicUnit=on
  ShowStringInMatlabConsole1 : MATLAB Function  TreatAsAtomicUnit=on
  WatchdogTimeout_ms : Constant  Value=500
  error_ : Concatenate  NumInputs=1
  isCabinetBlueButtonPressed_ : Concatenate  NumInputs=1
  isInitOk_ : Concatenate  NumInputs=1
  isMotorsOk_ : Concatenate  NumInputs=1
  isPatientDefined_ : Concatenate  NumInputs=1
  isTreadmillEmpty_ : Concatenate  NumInputs=1
  llcState : Display  Commented=on
      settings: AttributesFormatString=%<Tag>
  llcState_ : Concatenate  NumInputs=1
  ~Debug : Subsystem
      mask Display: disp('')
  Error : Outport
  LopesStatus : Outport  Port=2
  wires:
  AnyMessageWasReceived/1(Out1) -> GenerateString/4(AnyMessageWasReceivedByLLC)
  WatchdogTimeout_ms/1 -> GenerateString/3(WatchdogTimeout_ms)
  Ground/1 -> GenerateString/2(SegmentInertia)
  PreRecv/1 -> ShowStringInMatlabConsole1/3(pre)
  LLCReceiveUDPChannel1/2 -> ShowStringInMatlabConsole1/2(len), ParseString/2(s_len)
  LLCReceiveUDPChannel1/1 -> ShowStringInMatlabConsole1/1(stringArray), ParseString/1(s)
  PreSend/1 -> ShowStringInMatlabConsole/3(pre)
  Decimation/1 -> Logical Operator/2, GenerateString/Enable, LLCSendUDPChannel1/Enable
  ParseString/4(isInitOk) -> isInitOk_/1
  ParseString/7(isPatientDefined) -> isPatientDefined_/1
  ParseString/1(isParseException) -> AnyMessageWasReceived/1(In1), ErrorDisplay/1, error_/1
  ParseString/5(isMotorsOk) -> isMotorsOk_/1
  ParseString/2(llcState) -> llcState_/1
  ParseString/6(isTreadmillEmpty) -> isTreadmillEmpty_/1
  isPatientDefined_/1 -> Bus Creator/6  "isPatientDefined"
  isTreadmillEmpty_/1 -> Bus Creator/5  "isTreadmillEmpty"
  Bus Creator/1 -> LopesStatus/1
  isInitOk_/1 -> Bus Creator/3  "isInitOk"
  llcState_/1 -> llcState/1, Bus Creator/1  "llcState"
  isMotorsOk_/1 -> Bus Creator/4  "isMotorsOk"
  isCabinetBlueButtonPressed_/1 -> Bus Creator/2  "isCabinetBlueButtonPressed"
  GenerateString/2(s_len) -> LLCSendUDPChannel1/2, ShowStringInMatlabConsole/2(len)
  GenerateString/1(s) -> LLCSendUDPChannel1/1, ShowStringInMatlabConsole/1(stringArray)
  DesiredState/1 -> GenerateString/1(DesiredState)
  EnableDebugStringsInMatlab/1 -> Logical Operator1/1, Logical Operator/1
  Logical Operator/1 -> ShowStringInMatlabConsole/4(enable)
  One/1 -> LLCReceiveUDPChannel1/Enable, Logical Operator1/2, ParseString/Enable
  ParseString/3(isBlueCabinetButtonPressed) -> isCabinetBlueButtonPressed_/1
  Logical Operator1/1 -> ShowStringInMatlabConsole1/4(enable)
  error_/1 -> Error/1

== system LopesDevelopmentLibrary/Robot control blocks/RS232SyncBox ==
  note: You can use this block to send or receive (sync) pulses using the second RS232
      | (on the silver embedded PC's, this is the RS232 on the side where also keyboard
      | and network connectors are). This block was made to work together with the Lopes Sync Box.
      |
      | The input isSend determines the behaviour of this block:
      |
      | isSend==True (nonzero):
      | The system will send the (bool-typecast) of In to the DTR line of the RS232.
      | The output Out is made equal to In (such that, both for sending and receiving, Out reflects the sync pulse).
      |
      | isSend==False (zero):
      | The system sets the DTR and RTS such that the Sync box is configured for input;
      | then the output Out is set to what is coming in on the CTS input of the RS232. The value
      | of input In is ignored.
      |
      | This block was designed to be used with the Lopes-Sync Box. This box was constructed such
      | that for using the input on the box, DTR should be 0 and RTS should be 1.
  isSend : Inport
  In : Inport  Port=2
  Compare To Zero1 : simulink/Logic and Bit Operations/Compare To Zero  relop=~=  OutDataTypeStr=boolean
  DTR_Read : Constant  Value=0
  DTR_Send : DataTypeConversion  OutDataTypeStr=double
  Modem Control : xpcseriallib/Mainboard/Modem Control  rts=on  dtr=on  config=Com2  addr=0x3f8
  Modem Status : xpcseriallib/Mainboard/Modem Status  cts=on  dsr=off  ring=off  dcd=off  sampletime=HLCParams.ts  config=Com2  addr=0x3f8
  RTS_Read : Constant
  RTS_Send : Constant  Value=0
  Switch : Switch  Criteria=u2 ~= 0
  Switch1 : Switch  Criteria=u2 ~= 0
  Switch2 : Switch  Criteria=u2 ~= 0
  Out : Outport
  wires:
  isSend/1 -> Switch/2, Switch2/2, Switch1/2
  DTR_Send/1 -> Switch/1, Switch2/1
  Modem Status/1 -> Switch/3
  Switch/1 -> Out/1
  In/1 -> Compare To Zero1/1
  Switch2/1 -> Modem Control/2
  DTR_Read/1 -> Switch2/3
  Compare To Zero1/1 -> DTR_Send/1
  Switch1/1 -> Modem Control/1
  RTS_Send/1 -> Switch1/1
  RTS_Read/1 -> Switch1/3

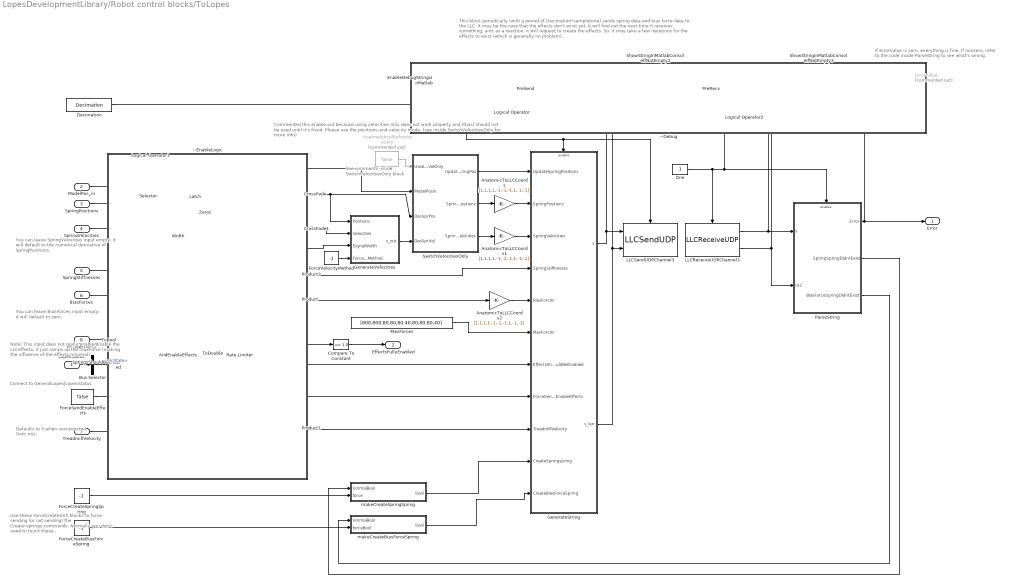
== system LopesDevelopmentLibrary/Robot control blocks/ToLopes ==
  note: You can leave BiasForces
      | input empty; it will default to zero.
  note: This block periodically (with a period of Decimation*sampletime) sends spring data and bias force
      | data to the LLC.
      | It may be the case that the effects don't exist yet. It will find out the next time it receives something, and,
      | as a reaction, it will request to create the effects. So, it may take a few iterations for the effects
      | to exist (which is generally no problem).
  note: If ErrorValue is zero, everything is fine. If nonzero,
      | refer to the code inside ParseString to see
      | what's wrong.
  note: Use these ForceCreateXXX
      | blocks to force sending (or not sending)
      | the Create-springs-commands.
      | Normally you don't need to touch these..
  note: You can leave SpringVelocities
      | input empty; it will default to the
      | numerical derivative of SpringPositions.
  note: Note: This input does not really enable/disable
      | the LLCeffects; it just ramps up the maxForce
      | (making the influence of the effects minimal)
  note: Connect to GeneralLopes|LopesStatus
  note: Defaults to 0 when unconnected.
      | Unit: m/s.
  note: See comments inside
      | SwitchVelocitiesOnly block
  note: Commented this enable out because using velocities only does not work properly and (thus) should not be used until it's fixed. Please use the positions-and-velocity mode. (see inside SwitchVelocitiesOnly for more info)
  LopesStatus : Inport
  ModelPos_in : Inport  Port=2
  SpringPositions : Inport  Port=3
  SpringVelocities : Inport  Port=4
  SpringStiffnesses : Inport  Port=5
  BiasForces : Inport  Port=6
  TreadmillVelocity : Inport  Port=7
  EnableEffects : Inport  Port=8
  AnatomicToLLCCoords : Gain  Gain=[1,1,1,1,-1,-1,-1,1,-1,-1]
  AnatomicToLLCCoords1 : Gain  Gain=[1,1,1,1,-1,-1,-1,1,-1,-1]
  AnatomicToLLCCoords2 : Gain  Gain=[1,1,1,1,-1,-1,-1,1,-1,-1]
  AndEnableEffects : Logic  AllPortsSameDT=off  OutDataTypeStr=boolean
  Bus Selector : BusSelector  OutputSignals=llcState
  Compare To Constant : simulink/Logic and Bit Operations/Compare To Constant  relop===  const=1.0  OutDataTypeStr=boolean
  CrossFade : Subsystem
  CrossFade1 : Subsystem
  Decimation : LopesDevelopmentLibrary/Various/Decimation
  EnableDebugStringsInMatlab : Constant  Value=0  OutDataTypeStr=double
      settings: OpenFcn=|
      | b = get_param(gcb,'value');
      | if (strcmp(b,'1')),
      |   set_param (gcb,'value','0');
      | else
      |   set_param(gcb,'value','1');
      | end;
  ErrorValue : Display  Commented=on
  ForceCreateBiasForceSpring : Constant  Value=-1
  ForceCreateSpringSpring : Constant  Value=-1
  ForceSendEnableEffects : Constant  Value=false  OutDataTypeStr=boolean
      settings: OpenFcn=|
      | b = get_param(gcb,'value');
      | if (strcmp(b,'true')),
      |   set_param (gcb,'value','false');
      | else
      |   set_param(gcb,'value','true');
      | end;
  ForceVelocityMethod : Constant  Value=-1
  GenerateString : Subsystem
  GenerateVelocities : Subsystem
  LLCReceiveUDPChannel3 : LopesDevelopmentLibrary/BlocksForInternalUse/LLC Communication/LLCReceiveUDP  port=LopesParams.Communication.channel3ReceivePort
  LLCSendUDPChannel3 : LopesDevelopmentLibrary/BlocksForInternalUse/LLC Communication/LLCSendUDP  port=LopesParams.Communication.channel3SendPort
  Latch : LopesDevelopmentLibrary/Various/Latch  ic=0
  Logical Operator : Logic  AllPortsSameDT=off  OutDataTypeStr=boolean
  Logical Operator1 : Logic  Operator=NOT  AllPortsSameDT=off  OutDataTypeStr=boolean
  Logical Operator2 : Logic  AllPortsSameDT=off  OutDataTypeStr=boolean
  MaxForces : Constant  Value=[800,800,80,80,80,40,80,80,80,40]
  One : Constant
  ParseString : Subsystem
  PreRecv : Constant  Value=uint8(['ToLopesRecv: '])
  PreSend : Constant  Value=uint8(['ToLopesSend: '])
  Product : Product  RndMeth=Zero
  Product1 : Product  RndMeth=Zero
  Product3 : Product  RndMeth=Zero
  Rate Limiter : RateLimiter  RisingSlewLimit=0.2  FallingSlewLimit=-inf  SampleTimeMode=inherited
  Selector : Selector  InputPortWidth=13  IndexOptions=Index vector (dialog)  Indices=[1:10]  OutputSizes=1
  ShowStringInMatlabConsoleIfNotEmpty2 : MATLAB Function  TreatAsAtomicUnit=on
  ShowStringInMatlabConsoleIfNotEmpty3 : MATLAB Function  TreatAsAtomicUnit=on
  SpringsShouldBeEnabled : LopesDevelopmentLibrary/Various/CompareAny  values=[4,5]
  SwitchVelocitiesOnly : Subsystem
  ToBool : DataTypeConversion  OutDataTypeStr=boolean
  ToDouble : DataTypeConversion  OutDataTypeStr=double
  UseAnalyticalVelocitiesOnly : Constant  Commented=on  Value=false  OutDataTypeStr=boolean
      settings: OpenFcn=|
      | b = get_param(gcb,'value');
      | if (strcmp(b,'true')),
      |   set_param (gcb,'value','false');
      | else
      |   set_param(gcb,'value','true');
      | end;
  Width : Width
  Zeros : Constant  Value=zeros(1,10)
  makeCreateBiasForceSpring : MATLAB Function  TreatAsAtomicUnit=on
  makeCreateSpringSpring : MATLAB Function  TreatAsAtomicUnit=on
  ~Debug : Subsystem
      mask Display: disp('')
  ~EnableLogic : Subsystem
  Error : Outport
  EffectsFullyEnabled : Outport  Port=2
  wires:
  AnatomicToLLCCoords1/1 -> GenerateString/3(SpringVelocities)
  UseAnalyticalVelocitiesOnly/1 -> SwitchVelocitiesOnly/1(UseAnalVelOnly)
  GenerateVelocities/1(v_out) -> SwitchVelocitiesOnly/4(DesSprVel)
  SwitchVelocitiesOnly/3(SpringVelocities) -> AnatomicToLLCCoords1/1
  SwitchVelocitiesOnly/1(UpdateSpringPos) -> GenerateString/1(UpdateSpringPositions)
  Product1/1 -> GenerateString/9(TreadmillVelocity)
  Compare To Constant/1 -> EffectsFullyEnabled/1
  AnatomicToLLCCoords2/1 -> GenerateString/5(BiasForces)
  ToBool/1 -> AndEnableEffects/1
  Selector/1 -> Latch/1, SwitchVelocitiesOnly/2(ModelPosIn)
  Latch/1 -> CrossFade/1(In1)
  Logical Operator1/1 -> Latch/Enable
  Zeros/1 -> CrossFade1/1(In1)
  ModelPos_in/1 -> Selector/1
  TreadmillVelocity/1 -> Product1/2
  EnableEffects/1 -> ToBool/1
  AndEnableEffects/1 -> ToDouble/1, Product3/2, Logical Operator1/1
  Width/1 -> GenerateVelocities/3(SignalWidth)
  CrossFade1/1(Out) -> GenerateVelocities/2(Velocities)
  ForceVelocityMethod/1 -> GenerateVelocities/4(ForceVelocityMethod)
  SpringVelocities/1 -> Width/1, CrossFade1/2(In2)
  Product/1 -> AnatomicToLLCCoords2/1
  CrossFade/1(Out) -> SwitchVelocitiesOnly/3(DesSprPos), GenerateVelocities/1(Positions)
  SpringsShouldBeEnabled/1 -> GenerateString/7(EffectsShouldBeEnabled), AndEnableEffects/2
  MaxForces/1 -> GenerateString/6(MaxForces)
  ToDouble/1 -> Rate Limiter/1
  Bus Selector/1 -> SpringsShouldBeEnabled/1  "<llcState>"
  BiasForces/1 -> Product/1
  Rate Limiter/1 -> Compare To Constant/1, Product1/1, Product/2, CrossFade/3(AmountIn2), CrossFade1/3(AmountIn2)
  ForceSendEnableEffects/1 -> GenerateString/8(ForceSendEnableEffects)
  LopesStatus/1 -> Bus Selector/1
  ParseString/1(Error) -> Error/1, ErrorValue/1
  ParseString/2(SpringSpringDidntExist) -> makeCreateSpringSpring/1(normalBool)
  ParseString/3(BiasForceSpringDidntExist) -> makeCreateBiasForceSpring/1(normalBool)
  makeCreateBiasForceSpring/1(bool) -> GenerateString/11(CreateBiasForceSpring)
  makeCreateSpringSpring/1(bool) -> GenerateString/10(CreateSpringspring)
  SpringPositions/1 -> CrossFade/2(In2)
  GenerateString/2(s_len) -> LLCSendUDPChannel3/2, ShowStringInMatlabConsoleIfNotEmpty2/2(len)
  GenerateString/1(s) -> LLCSendUDPChannel3/1, ShowStringInMatlabConsoleIfNotEmpty2/1(stringArray)
  ForceCreateSpringSpring/1 -> makeCreateSpringSpring/2(force)
  ForceCreateBiasForceSpring/1 -> makeCreateBiasForceSpring/2(forceBool)
  PreRecv/1 -> ShowStringInMatlabConsoleIfNotEmpty3/3(pre)
  LLCReceiveUDPChannel3/1 -> ParseString/1(s), ShowStringInMatlabConsoleIfNotEmpty3/1(stringArray)
  LLCReceiveUDPChannel3/2 -> ShowStringInMatlabConsoleIfNotEmpty3/2(len), ParseString/2(In2)
  Decimation/1 -> Logical Operator/2, GenerateString/Enable, LLCSendUDPChannel3/Enable
  PreSend/1 -> ShowStringInMatlabConsoleIfNotEmpty2/3(pre)
  EnableDebugStringsInMatlab/1 -> Logical Operator2/1, Logical Operator/1
  Logical Operator/1 -> ShowStringInMatlabConsoleIfNotEmpty2/4(enable)
  One/1 -> Logical Operator2/2, ParseString/Enable, LLCReceiveUDPChannel3/Enable
  Logical Operator2/1 -> ShowStringInMatlabConsoleIfNotEmpty3/4(enable)
  SpringStiffnesses/1 -> Product3/1
  SwitchVelocitiesOnly/2(SpringPositions) -> AnatomicToLLCCoords/1
  AnatomicToLLCCoords/1 -> GenerateString/2(SpringPositions)
  Product3/1 -> GenerateString/4(SpringStiffnesses)
